simulink model "fading_filter"  (R2020b)
settings: Solver=VariableStepAuto  StartTime=0.0  StopTime=10  RelTol=1e-3
model workspace (MAT data in the model file):
  variance = 10
undefined symbols (not defined in the file): Ts
libraries: simulink x3
settings Model: SimulationMode=rapid-accelerator  EnablePacing=on  Creator=stefano  LastModifiedBy=stefano

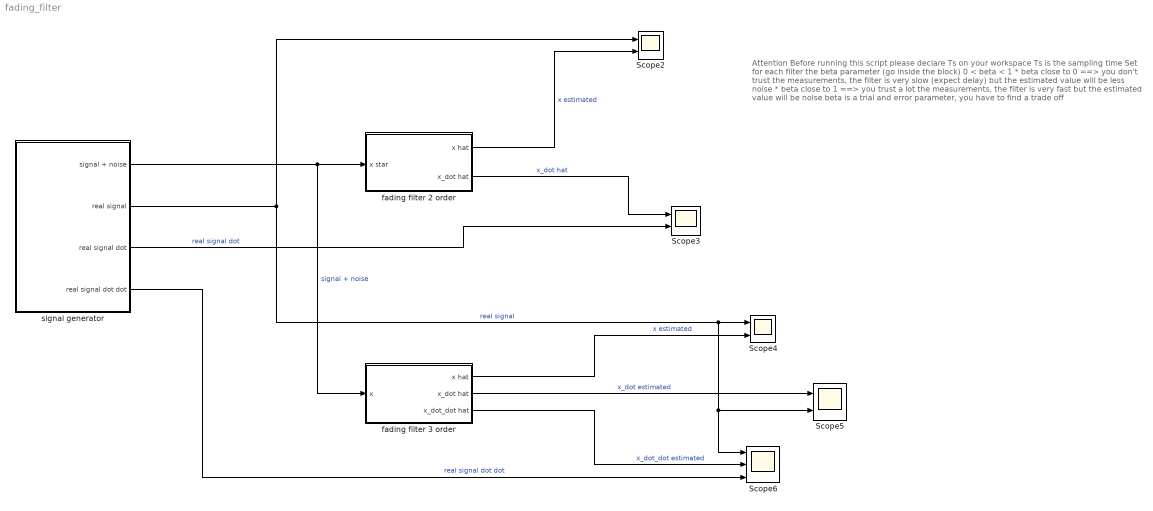
== system fading_filter ==
  note: Attention
      |
      | Before running this script please declare Ts on your workspace
      | Ts is the sampling time
      |
      | Set for each filter the beta parameter (go inside the block)
      |
      | 0 < beta < 1
      |
      | * beta close to 0 ==> you don't trust the measurements, the filter is very slow (expect delay) but the estimated value will be less noise
      | * beta close to 1 ==> you trust a lot the measurements, the filter is very fast but the estimated value will be noise
      |
      | beta is a trial and error parameter, you have to find a trade off
  Scope{2..5} (4 alike) : Scope  NumInputPorts=2
  Scope6 : Scope  NumInputPorts=3
  fading filter 2 order : Subsystem
  fading filter 3 order : Subsystem
  "signal generator " : Subsystem
  wires:
  "signal generator "/1(signal + noise) -> fading filter 2 order/1(x star), fading filter 3 order/1(x)  "signal + noise"
  fading filter 2 order/1(x hat) -> Scope2/2  "x estimated"
  fading filter 2 order/2(x_dot hat) -> Scope3/1  "x_dot hat"
  "signal generator "/2(real signal) -> Scope2/1, Scope6/1, Scope5/2, Scope4/1  "real signal"
  fading filter 3 order/1(x hat) -> Scope4/2  "x estimated"
  fading filter 3 order/2(x_dot hat) -> Scope5/1  "x_dot estimated"
  fading filter 3 order/3(x_dot_dot hat) -> Scope6/2  "x_dot_dot estimated"
  "signal generator "/3(real signal dot) -> Scope3/2  "real signal dot"
  "signal generator "/4(real signal dot dot) -> Scope6/3  "real signal dot dot"

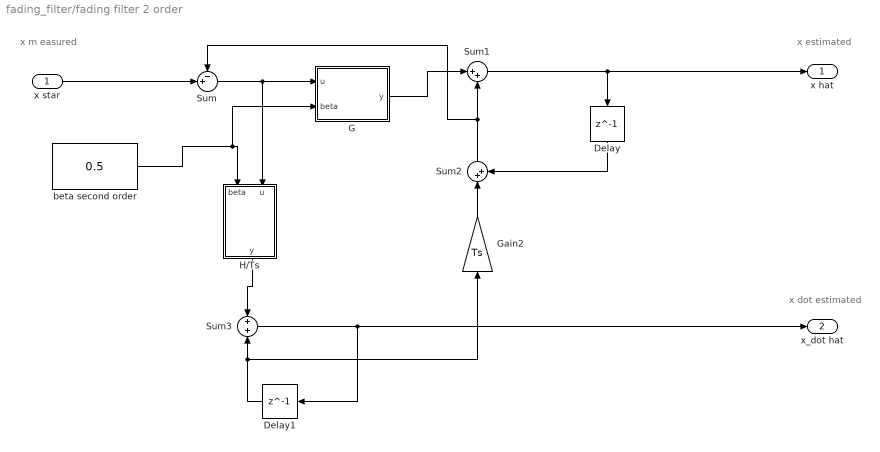
== system fading_filter/fading filter 2 order ==
  note: x dot estimated
  note: x m easured
  note: x estimated
  x star : Inport
  Delay : Delay  DelayLength=1
  Delay1 : Delay  DelayLength=1
  G : MATLAB Function  TreatAsAtomicUnit=on
  Gain2 : Gain  Gain=Ts
  H/Ts : MATLAB Function  TreatAsAtomicUnit=on
  Sum : Sum  Inputs=-+|
  Sum1 : Sum  Inputs=|++
  Sum2 : Sum  Inputs=|++
  Sum3 : Sum  Inputs=+|+
  beta second order : Constant  Value=0.5  OutDataTypeStr=Inherit: Inherit via back propagation
  x hat : Outport
  x_dot hat : Outport  Port=2
  wires:
  H/Ts/1(y) -> Sum3/1
  Sum2/1 -> Sum/1, Sum1/2
  Sum3/1 -> x_dot hat/1, Delay1/1
  Sum1/1 -> x hat/1, Delay/1
  Delay/1 -> Sum2/2
  Delay1/1 -> Gain2/1, Sum3/2
  Gain2/1 -> Sum2/1
  G/1(y) -> Sum1/1
  x star/1 -> Sum/2
  Sum/1 -> H/Ts/2(u), G/1(u)
  beta second order/1 -> G/2(beta), H/Ts/1(beta)

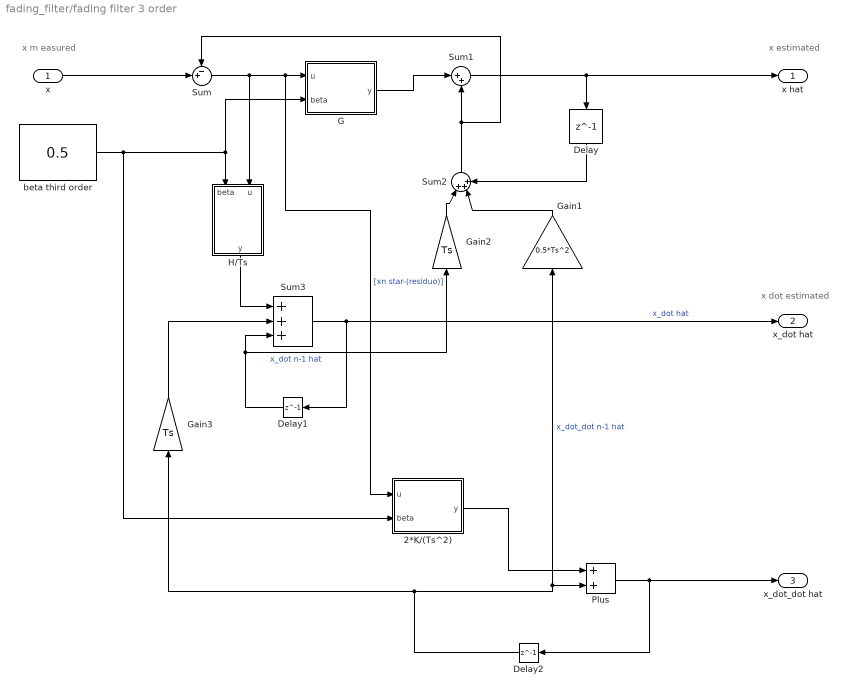
== system fading_filter/fading filter 3 order ==
  note: x dot estimated
  note: x m easured
  note: x estimated
  x : Inport
  2*K/(Ts^2) : MATLAB Function  TreatAsAtomicUnit=on
  Delay : Delay  DelayLength=1
  Delay1 : Delay  DelayLength=1
  Delay2 : Delay  DelayLength=1
  G : MATLAB Function  TreatAsAtomicUnit=on
  Gain1 : Gain  Gain=0.5*Ts^2
  Gain2 : Gain  Gain=Ts
  Gain3 : Gain  Gain=Ts
  H/Ts : MATLAB Function  TreatAsAtomicUnit=on
  Plus : Sum
  Sum : Sum  Inputs=-+|
  Sum1 : Sum  Inputs=|++
  Sum2 : Sum  Inputs=|+++
  Sum3 : Sum  Inputs=+++
  beta third order : Constant  Value=0.5  OutDataTypeStr=Inherit: Inherit via back propagation
  x hat : Outport
  x_dot hat : Outport  Port=2
  x_dot_dot hat : Outport  Port=3
  wires:
  H/Ts/1(y) -> Sum3/1
  Sum2/1 -> Sum/1, Sum1/2
  Sum3/1 -> Delay1/1, x_dot hat/1  "x_dot hat"
  Sum1/1 -> x hat/1, Delay/1
  Delay/1 -> Sum2/3
  Delay1/1 -> Sum3/3, Gain2/1  "x_dot n-1 hat"
  Gain2/1 -> Sum2/1
  G/1(y) -> Sum1/1
  x/1 -> Sum/2
  Sum/1 -> 2*K/(Ts^2)/1(u), G/1(u), H/Ts/2(u)  "[xn star-(residuo)]"
  beta third order/1 -> 2*K/(Ts^2)/2(beta), H/Ts/1(beta), G/2(beta)
  Gain1/1 -> Sum2/2
  Delay2/1 -> Plus/2, Gain1/1, Gain3/1  "x_dot_dot n-1 hat"
  Plus/1 -> x_dot_dot hat/1, Delay2/1
  Gain3/1 -> Sum3/2
  2*K/(Ts^2)/1(y) -> Plus/1

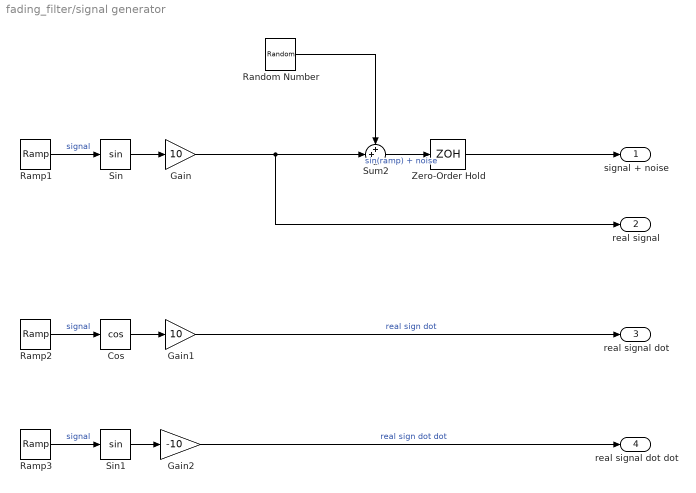
== system fading_filter/signal generator  ==
  Cos : Trigonometry  Operator=cos
  Gain : Gain  Gain=10
  Gain1 : Gain  Gain=10
  Gain2 : Gain  Gain=-10
  Ramp1 : simulink/Sources/Ramp  slope=1  start=0  InitialOutput=0
  Ramp2 : simulink/Sources/Ramp  slope=1  start=0  InitialOutput=0
  Ramp3 : simulink/Sources/Ramp  slope=1  start=0  InitialOutput=0
  Random Number : RandomNumber  Mean=0.1  Variance=2  SampleTime=Ts
  Sin : Trigonometry
  Sin1 : Trigonometry
  Sum2 : Sum  Inputs=++|
  Zero-Order Hold : ZeroOrderHold  SampleTime=Ts
  signal + noise : Outport
  real signal : Outport  Port=2
  real signal dot : Outport  Port=3
  real signal dot dot : Outport  Port=4
  wires:
  Random Number/1 -> Sum2/1
  Ramp1/1 -> Sin/1  "signal"
  Sin/1 -> Gain/1
  Sum2/1 -> Zero-Order Hold/1  "sin(ramp) + noise"
  Gain/1 -> real signal/1, Sum2/2
  Zero-Order Hold/1 -> signal + noise/1
  Cos/1 -> Gain1/1
  Ramp2/1 -> Cos/1  "signal"
  Ramp3/1 -> Sin1/1  "signal"
  Sin1/1 -> Gain2/1
  Gain1/1 -> real signal dot/1  "real sign dot"
  Gain2/1 -> real signal dot dot/1  "real sign dot dot"

== matlab function fading_filter/fading filter 2 order/G ==
  data: u input; y output; beta input
function y = fcn(u, beta)

y = u*(1-beta^2);

== matlab function fading_filter/fading filter 2 order/H//Ts ==
  data: beta input; u input; y output; Ts parameter
function y = fcn(beta, u, Ts)
y = ((1-beta)^2)*u/Ts;

== matlab function fading_filter/fading filter 3 order/H//Ts ==
  data: beta input; u input; y output; Ts parameter
function y = fcn(beta, u, Ts)
H=1.5*(1+beta)*(1-beta)^2;

y = u*H/Ts;

== matlab function fading_filter/fading filter 3 order/G ==
  data: u input; y output; beta input
function y = fcn(u, beta)

y = u*(1-beta^2);

== matlab function fading_filter/fading filter 3 order/2*K//(Ts^2) ==
  data: u input; y output; Ts parameter; beta input
function y = fcn(u, Ts, beta)
K = 0.5*((1-beta)^3);

y = u*2*K/(Ts^2);
